simulink model "l15_ex2_I"  (R2018b)
settings: Solver=ode45  StartTime=0.0  StopTime=30  MaxStep=1e-4  RelTol=1e-3  AbsTol=1e-3  EnableMultiTasking=on
values from neighbouring files (symbols this model uses):
  Ki = Ki_list(k)    [l15.m]    (also in l18.m = 5.65)
settings Model: Creator=Joe  LastModifiedBy=joema
settings SolverCC: AutoScaleAbsTol=off
settings DataIOCC: LimitDataPoints=on  SaveFormat=Array
settings OptimizationCC: LifeSpan=inf
settings DebuggingCC: UnderspecifiedInitializationDetection=Classic  MergeDetectMultiDrivingBlocksExec=none  LibraryContextMissingDiagnostic=none  SFUnexpectedBacktrackingDiag=warning  SFNoUnconditionalDefaultTransitionDiag=warning  SFExecutionAtInitializationDiag=none
settings HardwareCC: ProdBitPerPointer=32  ProdBitPerSizeT=32  ProdBitPerPtrDiffT=32  ProdLargestAtomicFloat=None  ProdIntDivRoundTo=Undefined  ProdEndianess=Unspecified  ProdWordSize=32  ProdHWDeviceType=32-bit Generic
settings ModelReferenceCC: PropagateSignalLabelsOutOfModel=off
settings SFSimCC: SimUseLocalCustomCode=off
settings RTWCC: RTWUseLocalCustomCode=off
settings CodeAppCC: StateflowObjectComments=on
settings GRTTargetCC: TargetLangStandard=C89/C90 (ANSI)  GeneratePreprocessorConditionals=Disable all
settings ConfigComp: CovMetricSettings=dw  CovHtmlReporting=on  CovSaveCumulativeToWorkspaceVar=on  CovSaveSingleToWorkspaceVar=on  CovExternalEMLEnable=off  CovSFcnEnable=off

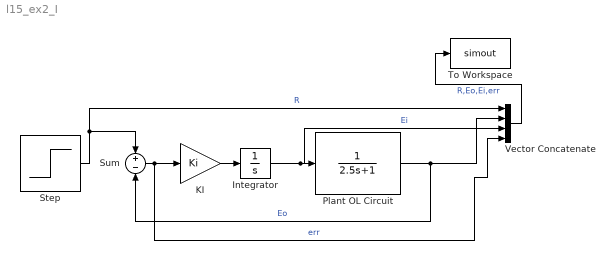
== system l15_ex2_I ==
  Integrator : Integrator
  KI : Gain  Gain=Ki
  Plant OL Circuit : TransferFcn  Denominator=[2.5 1]
  Step : Step  Time=0  After=5  SampleTime=0
  Sum : Sum  Inputs=+-
  To Workspace : ToWorkspace  VariableName=simout  SaveFormat=Timeseries  SampleTime=-1
  Vector Concatenate : Concatenate  NumInputs=4
  wires:
  Step/1 -> Vector Concatenate/1, Sum/1  "R"
  Sum/1 -> Vector Concatenate/4, KI/1  "err"
  KI/1 -> Integrator/1
  Plant OL Circuit/1 -> Vector Concatenate/2, Sum/2  "Eo"
  Integrator/1 -> Vector Concatenate/3, Plant OL Circuit/1  "Ei"
  Vector Concatenate/1 -> To Workspace/1  "R,Eo,Ei,err"
